simulink model "satellite_ADCS_detumbling_simulation_reaction_wheels"  (R2022b)
settings: Solver=FixedStepAuto  StartTime=t0  StopTime=T_o  FixedStep=0.1  RelTol=1e-9  AbsTol=1e-9
values from neighbouring files (symbols this model uses):
  A0 = Af    [satellite_ADCS_LEOP_simulation.m]
  a0 = [adx0 ady0 adz0 ax0 ay0 az0]    [satellite_ADCS_LEOP_simulation.m]
  A_sb_1 = [999.999999992226e-003    3.46376307675883e-006   -1.88420189887425e-006 ... (first row only)    [satellite_ADCS_LEOP_simulation.m]
  A_sb_2 = [999.999999948501e-003   -10.1488410044293e-006   -22.0178875132149e-012 ... (first row only)    [satellite_ADCS_LEOP_simulation.m]
  A_sb_3 = [999.999999975613e-003   -46.6812699606578e-012    6.98384920637069e-006 ... (first row only)    [satellite_ADCS_LEOP_simulation.m]
  Ac = [0 (1-Ky)*n 0 -Ky*n^2 0 0 ... (first row only)    [satellite_ADCS_LEOP_simulation.m]
  alphaG_0 = pi/1.5    (= 2.09439510239)    [satellite_ADCS_LEOP_simulation.m]
  ARW = [0 0; 1 0; 0 1]    [satellite_ADCS_LEOP_simulation.m]
  Bc = [J^-1; zeros(3,3)]    [satellite_ADCS_LEOP_simulation.m]
  Cc = [0 0 0 1 0 0 ... (first row only)    [satellite_ADCS_LEOP_simulation.m]
  Dc = zeros(3,3)    [satellite_ADCS_LEOP_simulation.m]
  E = 1    [satellite_ADCS_LEOP_simulation.m]
  F = 1e-3    (= 0.001)    [satellite_ADCS_LEOP_simulation.m]
  FOV = deg2rad(21.7)    [satellite_ADCS_LEOP_simulation.m]
  g_nm = S_matrix.*g_coefficients    [satellite_ADCS_LEOP_simulation.m]
  h_nm = S_matrix.*h_coefficients    [satellite_ADCS_LEOP_simulation.m]
  Irw = 80e-6    (= 8e-05)    [satellite_ADCS_LEOP_simulation.m]
  J = diag([Ix,Iy,Iz])    [satellite_ADCS_LEOP_simulation.m]
  J2 = 1.082e-3    (= 0.001082)    [satellite_ADCS_LEOP_simulation.m]
  K = lqry(SC,Qc,Rc)    [satellite_ADCS_LEOP_simulation.m]
  K_matrix = zeros(5,6)    [satellite_ADCS_LEOP_simulation.m]
  kep = [a e i OM om thf]    [satellite_ADCS_LEOP_simulation.m]
  L = Lt'    [satellite_ADCS_LEOP_simulation.m]
  LL = 1e-5    (= 1e-05)    [satellite_ADCS_LEOP_simulation.m]
  m = [0.37 0.32 0.28]    [satellite_ADCS_LEOP_simulation.m]
  mu = astroConstants(13)    [satellite_ADCS_LEOP_simulation.m]
  n = sqrt(mu/(a^3))    [satellite_ADCS_LEOP_simulation.m]
  n_sun = 2*pi/T_y    (= 1.99238499086e-07)    [satellite_ADCS_LEOP_simulation.m]
  omega_e = 2*pi/T_e    (= 7.27220521664e-05)    [satellite_ADCS_LEOP_simulation.m]
  P00 = 1    [satellite_ADCS_LEOP_simulation.m]
  pARW = pinv(ARW)    [satellite_ADCS_LEOP_simulation.m]
  pRRW = pinv(RRW)    [satellite_ADCS_LEOP_simulation.m]
  RRW = [R(:,3) R(:,6)]    [satellite_ADCS_LEOP_simulation.m]
  rt = astroConstants(23)    [satellite_ADCS_LEOP_simulation.m]
  S = S'    [satellite_ADCS_LEOP_simulation.m]
  sensor_noise = deg2rad(50/3600)    [satellite_ADCS_LEOP_simulation.m]
  sensor_sample_time = 1    [satellite_ADCS_LEOP_simulation.m]
  t0 = tf    (= 3200)    [satellite_ADCS_LEOP_simulation.m]
  T_o = 2*pi/n    [satellite_ADCS_LEOP_simulation.m]
  Te = 0.03    [satellite_ADCS_LEOP_simulation.m]
  Tp = [999.999926226686e-003    355.891478141766e-006   -144.526391847740e-006 ... (first row only)    [satellite_ADCS_LEOP_simulation.m]
  UL = 1e-4    (= 0.0001)    [satellite_ADCS_LEOP_simulation.m]
  w0 = wf    [satellite_ADCS_LEOP_simulation.m]
libraries: matrix_library x9, vrlib x3, sharedutil x2, aerolibutil x2
(part 1 of 3)
settings Model: Creator=user  LastModifiedBy=mutti
settings SolverCC: ZeroCrossAlgorithm=Adaptive
settings DebuggingCC: IgnoredZcDiagnostic=none  UnconnectedInputMsg=warning  UnconnectedOutputMsg=warning  UnconnectedLineMsg=warning
settings ModelReferenceCC: EnableRefExpFcnMdlSchedulingChecks=on
settings RTWCC: DLArmComputeVersion=19.05

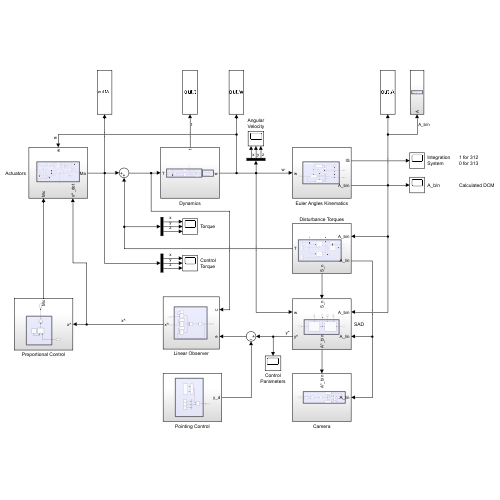
[thumbnail: Simulink's stored preview of the top-level diagram]
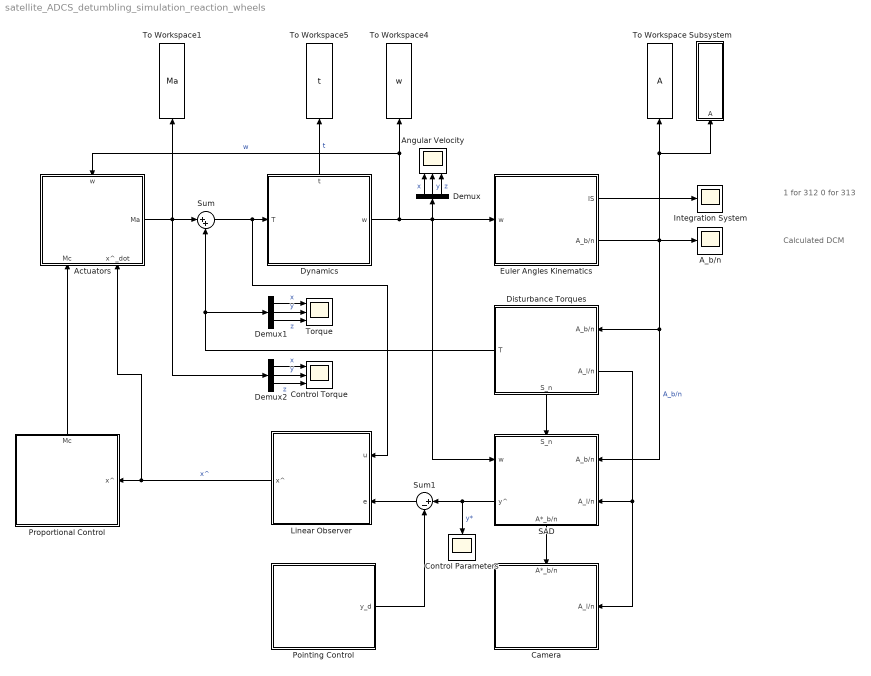
== system satellite_ADCS_detumbling_simulation_reaction_wheels ==
  note: Calculated DCM
  note: 1 for 312
      | 0 for 313
  A_b/n : Scope
  Actuators : Subsystem
      settings: PortSchema="{\"entries\":[{\"content\":{\"sides\":[{\"content\":{\"connectorIds\":[]},\"type\":\"ConnectorPlacement.EquallySpacedRectSide\",\"uuid\":\"a0a9569f-fefa-4f19-b459-3352d21c4e78\"},{\"content\":{\"connectorIds\":[\"Out1\"],\"side\":\"RIGHT\"},\"type\":\"ConnectorPlacement.EquallySpacedRectSide\",\"uuid\":\"2ed4db34-f6b5-4db4-9643-fbe8b2d4c52e\"},{\"content\":{\"connectorIds\":[\"In1\"],\"side\":\"TOP\"},\"type\":\"ConnectorPlacement.EquallySpacedRectSide\",\"uuid\":\"588bf8a5-5948-433a-b01f-23f1c7f2767b\"},{\"content\":{\"connectorIds\":[\"In2\",\"In3\"],\"side\":\"BOTTOM\"},\"type\":\"ConnectorPlacement.EquallySpacedRectSide\",\"uuid\":\"74bf1768-e871-4852-aab7-12511eae1523\"}]},\"type\":\"ConnectorPlacement.EquallySpacedConnector\",\"uuid\":\"47f49737-05d9-4a9e-a53b-421c1f23d8ed\"}],\"packageUris\":[\"http://schema.mathworks.com/mf0/Connector/R2020b\"],\"version\":\"1.0\"}"
  Angular Velocity : Scope  NumInputPorts=3
  Camera : Subsystem
      settings: PortSchema="{\"entries\":[{\"content\":{\"sides\":[{\"content\":{\"connectorIds\":[]},\"type\":\"ConnectorPlacement.EquallySpacedRectSide\",\"uuid\":\"e0342758-6e9b-40ff-85f6-f597544b67fd\"},{\"content\":{\"connectorIds\":[\"In2\"],\"side\":\"RIGHT\"},\"type\":\"ConnectorPlacement.EquallySpacedRectSide\",\"uuid\":\"f1e7fd7c-e0fe-4b5c-979b-e210999abd13\"},{\"content\":{\"connectorIds\":[\"In1\"],\"side\":\"TOP\"},\"type\":\"ConnectorPlacement.EquallySpacedRectSide\",\"uuid\":\"d086a2d5-2a33-45d1-927e-e3365679e422\"}]},\"type\":\"ConnectorPlacement.EquallySpacedConnector\",\"uuid\":\"0e539776-2a37-4829-8b62-d03ad8f161c7\"}],\"packageUris\":[\"http://schema.mathworks.com/mf0/Connector/R2020b\"],\"version\":\"1.0\"}"
  Control Parameters : Scope
  Control Torque : Scope  NumInputPorts=3
  Demux : Demux  Outputs=3
  Demux1 : Demux  Outputs=3
  Demux2 : Demux  Outputs=3
  Disturbance Torques : Subsystem
      settings: PortSchema="{\"entries\":[{\"content\":{\"sides\":[{\"content\":{\"connectorIds\":[\"In1\",\"Out3\"]},\"type\":\"ConnectorPlacement.EquallySpacedRectSide\",\"uuid\":\"d8dbad7b-a4da-4329-8f6c-994df882582d\"},{\"content\":{\"connectorIds\":[\"Out1\"],\"side\":\"RIGHT\"},\"type\":\"ConnectorPlacement.EquallySpacedRectSide\",\"uuid\":\"71b72684-f507-4d89-9cb7-6797f090e973\"},{\"content\":{\"connectorIds\":[],\"side\":\"TOP\"},\"type\":\"ConnectorPlacement.EquallySpacedRectSide\",\"uuid\":\"b8ec4cb7-c2c1-48ba-a366-4a3a04a391cc\"},{\"content\":{\"connectorIds\":[\"Out2\"],\"side\":\"BOTTOM\"},\"type\":\"ConnectorPlacement.EquallySpacedRectSide\",\"uuid\":\"004aaa39-3140-479a-bdad-82dbff681ba0\"}]},\"type\":\"ConnectorPlacement.EquallySpacedConnector\",\"uuid\":\"ddc3df03-ef2b-49f6-b8e4-ebb938f47d6c\"}],\"packageUris\":[\"http://schema.mathworks.com/mf0/Connector/R2020b\"],\"version\":\"1.0\"}"
  Dynamics : Subsystem
      settings: PortSchema="{\"entries\":[{\"content\":{\"sides\":[{\"content\":{\"connectorIds\":[\"In1\"]},\"type\":\"ConnectorPlacement.EquallySpacedRectSide\",\"uuid\":\"e7b72fe9-4828-4452-a73c-2aaa17307ac7\"},{\"content\":{\"connectorIds\":[\"Out1\"],\"side\":\"RIGHT\"},\"type\":\"ConnectorPlacement.EquallySpacedRectSide\",\"uuid\":\"e84d647a-1118-4c7e-bc5c-dae15a42ae60\"},{\"content\":{\"connectorIds\":[\"Out2\"],\"side\":\"TOP\"},\"type\":\"ConnectorPlacement.EquallySpacedRectSide\",\"uuid\":\"569f1d88-6323-45de-8d4a-941f3a02b2f9\"}]},\"type\":\"ConnectorPlacement.EquallySpacedConnector\",\"uuid\":\"aa1e349e-a763-481c-95bf-6bf3ac91b468\"}],\"packageUris\":[\"http://schema.mathworks.com/mf0/Connector/R2020b\"],\"version\":\"1.0\"}"
  Euler Angles Kinematics : Subsystem
  Integration System : Scope
  Linear Observer : Subsystem
  Pointing Control : Subsystem
  Proportional Control : Subsystem
      settings: PortSchema="{\"entries\":[{\"content\":{\"sides\":[{\"content\":{\"connectorIds\":[]},\"type\":\"ConnectorPlacement.EquallySpacedRectSide\",\"uuid\":\"b55cb1e2-f8e3-4e70-b41f-1afef80754b6\"},{\"content\":{\"connectorIds\":[\"In1\"],\"side\":\"RIGHT\"},\"type\":\"ConnectorPlacement.EquallySpacedRectSide\",\"uuid\":\"efac30e1-3844-4796-88a6-2f6a0b4b5a1e\"},{\"content\":{\"connectorIds\":[\"Out1\"],\"side\":\"TOP\"},\"type\":\"ConnectorPlacement.EquallySpacedRectSide\",\"uuid\":\"03ef4747-b6ea-4759-bd62-b95959aa7b4f\"}]},\"type\":\"ConnectorPlacement.EquallySpacedConnector\",\"uuid\":\"ca8bc0e9-cee1-4f1e-ac68-a532e2ed0ced\"}],\"packageUris\":[\"http://schema.mathworks.com/mf0/Connector/R2020b\"],\"version\":\"1.0\"}"
  SAD : Subsystem
      settings: PortSchema="{\"entries\":[{\"content\":{\"sides\":[{\"content\":{\"connectorIds\":[\"In1\",\"Out2\"]},\"type\":\"ConnectorPlacement.EquallySpacedRectSide\",\"uuid\":\"4f277e89-d200-473f-af52-c9445afe2970\"},{\"content\":{\"connectorIds\":[\"In3\",\"In4\"],\"side\":\"RIGHT\"},\"type\":\"ConnectorPlacement.EquallySpacedRectSide\",\"uuid\":\"94984762-2a8a-4315-bbca-0599c057d803\"},{\"content\":{\"connectorIds\":[\"In2\"],\"side\":\"TOP\"},\"type\":\"ConnectorPlacement.EquallySpacedRectSide\",\"uuid\":\"7e735617-ddb2-4178-9919-23d54f0f435d\"},{\"content\":{\"connectorIds\":[\"Out1\"],\"side\":\"BOTTOM\"},\"type\":\"ConnectorPlacement.EquallySpacedRectSide\",\"uuid\":\"8618ad89-dd0b-4af6-bdfc-ad96cd4377bc\"}]},\"type\":\"ConnectorPlacement.EquallySpacedConnector\",\"uuid\":\"e5f6a8ae-b3bf-403b-9441-c8c91592678e\"}],\"packageUris\":[\"http://schema.mathworks.com/mf0/Connector/R2020b\"],\"version\":\"1.0\"}"
  Subsystem : Subsystem
  Sum : Sum  Inputs=|++
  Sum1 : Sum  Inputs=|+-
  To Workspace : ToWorkspace  VariableName=A  SampleTime=-1
  To Workspace1 : ToWorkspace  VariableName=Ma  SampleTime=-1
  To Workspace4 : ToWorkspace  VariableName=w  SampleTime=-1
  To Workspace5 : ToWorkspace  VariableName=t  SampleTime=-1
  Torque : Scope  NumInputPorts=3
  wires:
  Dynamics/2(t) -> To Workspace5/1  "t"
  Dynamics/1(w) -> Demux/1, SAD/1(w), Euler Angles Kinematics/1(w), To Workspace4/1, Actuators/1(w)  "w"
  Euler Angles Kinematics/2(A_b/n) -> SAD/3(A_b/n), Disturbance Torques/1(A_b/n), A_b/n/1, Subsystem/1(A), To Workspace/1  "A_b/n"
  Demux/3 -> Angular Velocity/3  "z"
  Demux/2 -> Angular Velocity/2  "y"
  Demux/1 -> Angular Velocity/1  "x"
  Disturbance Torques/1(T) -> Sum/2, Demux1/1
  Demux1/1 -> Torque/1  "x"
  Demux1/3 -> Torque/3  "z"
  Demux1/2 -> Torque/2  "y"
  Euler Angles Kinematics/1(IS) -> Integration System/1
  Disturbance Torques/3(A_l/n) -> Camera/2(A_l/n), SAD/4(A_l/n)
  Sum/1 -> Linear Observer/1(u), Dynamics/1(T)
  SAD/2(y^) -> Sum1/1, Control Parameters/1  "y*"
  Disturbance Torques/2(S_n) -> SAD/2(S_n)
  Linear Observer/1(x^) -> Actuators/3(x^_dot), Proportional Control/1(x^)  "x^"
  Demux2/2 -> Control Torque/2  "y"
  Demux2/3 -> Control Torque/3  "z"
  Demux2/1 -> Control Torque/1  "x"
  Actuators/1(Ma) -> Demux2/1, Sum/1, To Workspace1/1
  SAD/1(A*_b/n) -> Camera/1(A*_b/n)
  Sum1/1 -> Linear Observer/2(e)
  Pointing Control/1(y_d) -> Sum1/2
  Proportional Control/1(Mc) -> Actuators/2(Mc)

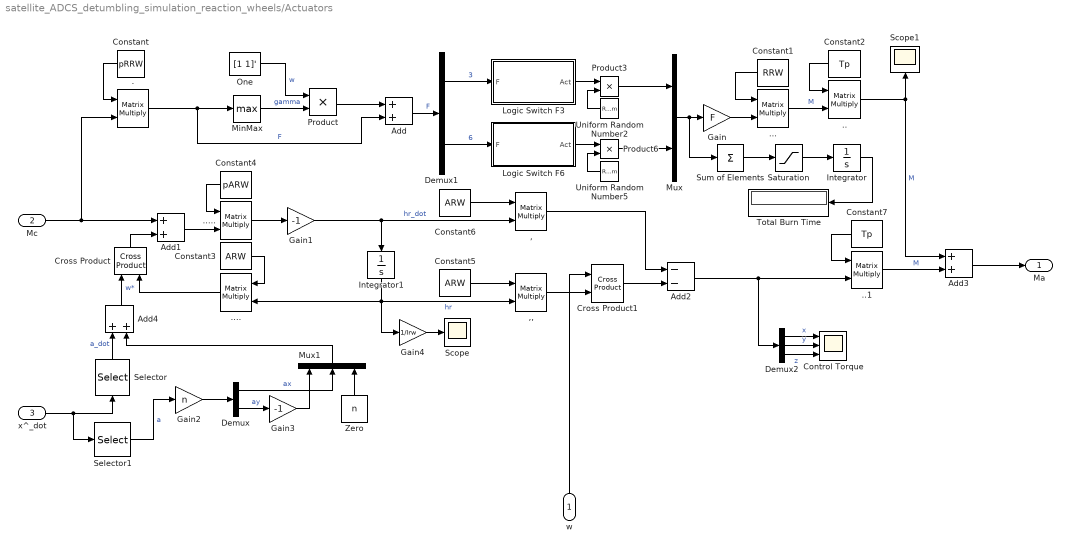
== system satellite_ADCS_detumbling_simulation_reaction_wheels/Actuators ==
  w : Inport
  Mc : Inport  Port=2
  x^_dot : Inport  Port=3
  , : Product  Multiplication=Matrix(*)
  ,, : Product  Multiplication=Matrix(*)
  . : Product  Multiplication=Matrix(*)
  .. : Product  Multiplication=Matrix(*)
  ... : Product  Multiplication=Matrix(*)
  .... : Product  Multiplication=Matrix(*)
  ..... : Product  Multiplication=Matrix(*)
  ..1 : Product  Multiplication=Matrix(*)
  Add{,1,3..4} (4 alike) : Sum
  Add2 : Sum  Inputs=--
  Constant : Constant  Value=pRRW
  Constant1 : Constant  Value=RRW
  Constant2 : Constant  Value=Tp
  Constant3 : Constant  Value=ARW
  Constant4 : Constant  Value=pARW
  Constant5 : Constant  Value=ARW
  Constant6 : Constant  Value=ARW
  Constant7 : Constant  Value=Tp
  Control Torque : Scope  NumInputPorts=3
  Cross Product : matrix_library/Cross Product
  Cross Product1 : matrix_library/Cross Product
  Demux : Demux  Outputs=2
  Demux1 : Demux  Outputs=2
  Demux2 : Demux  Outputs=3
  Gain : Gain  Gain=F
  Gain1 : Gain  Gain=-1
  Gain2 : Gain  Gain=n
  Gain3 : Gain  Gain=-1
  Gain4 : Gain  Gain=1/Irw
  Integrator : Integrator
  Integrator1 : Integrator  InitialCondition=[0 0]'
  Logic Switch F3 : Subsystem
  Logic Switch F6 : Subsystem
  MinMax : MinMax  Function=max
  Mux : Mux  Inputs=2
  Mux1 : Mux  Inputs=3
  One : Constant  Value=[1 1]'  OutDataTypeStr=Inherit: Inherit via back propagation
  Product : Product
  Product3 : Product
  Product6 : Product
  Saturation : Saturate  UpperLimit=1  LowerLimit=0
  Scope : Scope
  Scope1 : Scope
  Selector : Selector  InputPortWidth=6  IndexOptions=Index vector (dialog)  Indices=[1 2 3]  OutputSizes=1
  Selector1 : Selector  InputPortWidth=6  IndexOptions=Index vector (dialog)  Indices=[4 5]  OutputSizes=1
  Sum of Elements : Sum  Inputs=+
  Total Burn Time : Display
  Uniform Random Number2 : UniformRandomNumber  Minimum=1-Te  Maximum=1+Te  SampleTime=sensor_sample_time
  Uniform Random Number5 : UniformRandomNumber  Minimum=1-Te  Maximum=1+Te  SampleTime=sensor_sample_time
  Zero : Constant  Value=n  OutDataTypeStr=Inherit: Inherit via back propagation
  Ma : Outport
  wires:
  Gain4/1 -> Scope/1
  ..1/1 -> Add3/2  "M"
  Constant7/1 -> ..1/1
  Demux2/1 -> Control Torque/1  "x"
  Add2/1 -> ..1/2, Demux2/1
  Demux2/2 -> Control Torque/2  "y"
  Demux2/3 -> Control Torque/3  "z"
  Mux1/1 -> Add4/2
  Add4/1 -> Cross Product/1  "w*"
  Zero/1 -> Mux1/3
  Gain3/1 -> Mux1/1
  x^_dot/1 -> Selector1/1, Selector/1
  Gain2/1 -> Demux/1
  Demux/2 -> Gain3/1  "ay"
  Demux/1 -> Mux1/2  "ax"
  Selector1/1 -> Gain2/1  "a"
  Selector/1 -> Add4/1  "a_dot"
  Add3/1 -> Ma/1
  ,/1 -> Add2/1
  Cross Product1/1 -> Add2/2
  Constant6/1 -> ,/1
  ,,/1 -> Cross Product1/2
  Constant5/1 -> ,,/1
  w/1 -> Cross Product1/1
  Cross Product/1 -> Add1/2
  ..../1 -> Cross Product/2
  Gain1/1 -> ,/2, Integrator1/1  "hr_dot"
  ...../1 -> Gain1/1
  Constant4/1 -> ...../1
  Add1/1 -> ...../2
  Constant3/1 -> ..../1
  Integrator1/1 -> ..../2, ,,/2, Gain4/1  "hr"
  Constant2/1 -> ../1
  Constant1/1 -> .../1
  .../1 -> ../2  "M"
  Product3/1 -> Mux/1
  Product6/1 -> Mux/2
  Uniform Random Number5/1 -> Product6/2
  Uniform Random Number2/1 -> Product3/2
  Integrator/1 -> Total Burn Time/1
  Saturation/1 -> Integrator/1
  Sum of Elements/1 -> Saturation/1
  Gain/1 -> .../2
  Mux/1 -> Gain/1, Sum of Elements/1
  Logic Switch F3/1(Act) -> Product3/1
  Logic Switch F6/1(Act) -> Product6/1
  ../1 -> Scope1/1, Add3/1  "M"
  Demux1/1 -> Logic Switch F3/1(F)  "3"
  Demux1/2 -> Logic Switch F6/1(F)  "6"
  Add/1 -> Demux1/1  "F"
  Product/1 -> Add/1
  One/1 -> Product/1  "w"
  MinMax/1 -> Product/2  "gamma"
  ./1 -> Add/2, MinMax/1  "F"
  Mc/1 -> ./2, Add1/1
  Constant/1 -> ./1

== system satellite_ADCS_detumbling_simulation_reaction_wheels/Camera ==
  A*_b/n : Inport
  A_l/n : Inport  Port=2
  . : Product  Multiplication=Matrix(*)
  Asin : Trigonometry  Operator=asin
  Atan2 : Trigonometry  Operator=atan2
  Demux : Demux  Outputs=3
  Gain : Gain  Gain=-1
  Reshape : Reshape
  Reshape1 : Reshape
  Scope : Scope  NumInputPorts=2
  Selector : Selector  NumberOfDimensions=2  InputPortWidth=3  IndexOptions=Index vector (dialog),Index vector (dialog)  Indices=[1 2 3],1  OutputSizes=1,1
  To Workspace : ToWorkspace  VariableName=lat_lambda  SampleTime=-1
      settings: Save2DSignal=2-D array (concatenate along first dimension)
  To Workspace1 : ToWorkspace  VariableName=long_phi  SampleTime=-1
      settings: Save2DSignal=2-D array (concatenate along first dimension)
  Transpose : Math  Operator=transpose
  wires:
  A_l/n/1 -> Transpose/1
  A*_b/n/1 -> ./1
  ./1 -> Selector/1  "A_b/l"
  Selector/1 -> Demux/1  "x_b/l"
  Demux/3 -> Asin/1
  Asin/1 -> Scope/2, Reshape/1  "lat lambda"
  Demux/2 -> Atan2/1
  Demux/1 -> Atan2/2
  Atan2/1 -> Gain/1
  Transpose/1 -> ./2  "A_n/l"
  Gain/1 -> Scope/1, Reshape1/1  "long phi"
  Reshape/1 -> To Workspace/1
  Reshape1/1 -> To Workspace1/1

== system satellite_ADCS_detumbling_simulation_reaction_wheels/Disturbance Torques ==
  A_b/n : Inport
  Attitude Error : Subsystem
      settings: PortSchema="{\"entries\":[{\"content\":{\"sides\":[{\"content\":{\"connectorIds\":[\"In1\",\"Out1\"]},\"type\":\"ConnectorPlacement.EquallySpacedRectSide\",\"uuid\":\"42b76f21-72ca-4a81-86e8-c766a84eaf13\"},{\"content\":{\"connectorIds\":[],\"side\":\"RIGHT\"},\"type\":\"ConnectorPlacement.EquallySpacedRectSide\",\"uuid\":\"045cfb84-697d-470f-9812-3dd1de7d9dae\"},{\"content\":{\"connectorIds\":[],\"side\":\"TOP\"},\"type\":\"ConnectorPlacement.EquallySpacedRectSide\",\"uuid\":\"bb53017d-cb0a-420c-8e45-e706475f7b71\"},{\"content\":{\"connectorIds\":[\"In2\"],\"side\":\"BOTTOM\"},\"type\":\"ConnectorPlacement.EquallySpacedRectSide\",\"uuid\":\"54ff18d1-a59a-458c-93f1-94e0d804cb2b\"}]},\"type\":\"ConnectorPlacement.EquallySpacedConnector\",\"uuid\":\"29a17c75-6caa-44fa-8f21-b7e933b3095b\"}],\"packageUris\":[\"http://schema.mathworks.com/mf0/Connector/R2020b\"],\"version\":\"1.0\"}"
  GG Torque : Scope
  GGT : Subsystem
      settings: PortSchema="{\"entries\":[{\"content\":{\"sides\":[{\"content\":{\"connectorIds\":[]},\"type\":\"ConnectorPlacement.EquallySpacedRectSide\",\"uuid\":\"c87f4cc9-8c7a-4c3d-b61f-c042856a7ec9\"},{\"content\":{\"connectorIds\":[],\"side\":\"RIGHT\"},\"type\":\"ConnectorPlacement.EquallySpacedRectSide\",\"uuid\":\"826a080d-b2ad-4022-8511-2b74ea66cdbd\"},{\"content\":{\"connectorIds\":[\"Out1\",\"Out2\"],\"side\":\"TOP\"},\"type\":\"ConnectorPlacement.EquallySpacedRectSide\",\"uuid\":\"8ee238e0-7e27-4db5-8615-50d5a9b316be\"}]},\"type\":\"ConnectorPlacement.EquallySpacedConnector\",\"uuid\":\"2b8a1979-eb0c-41eb-af64-c98b651bcc5f\"}],\"packageUris\":[\"http://schema.mathworks.com/mf0/Connector/R2020b\"],\"version\":\"1.0\"}"
  Gravity Gradient Torque : Subsystem
  Local S/C Frame : Subsystem
      settings: PortSchema="{\"entries\":[{\"content\":{\"sides\":[{\"content\":{\"connectorIds\":[\"Out3\"]},\"type\":\"ConnectorPlacement.EquallySpacedRectSide\",\"uuid\":\"19c66f1b-1487-47a5-99ee-e01045e7a130\"},{\"content\":{\"connectorIds\":[\"Out1\"],\"side\":\"RIGHT\"},\"type\":\"ConnectorPlacement.EquallySpacedRectSide\",\"uuid\":\"23994730-2288-4426-9fea-174ee661e5cc\"},{\"content\":{\"connectorIds\":[\"Out2\"],\"side\":\"TOP\"},\"type\":\"ConnectorPlacement.EquallySpacedRectSide\",\"uuid\":\"3f4149a4-c086-47bf-a88a-6d224e7bd6a7\"}]},\"type\":\"ConnectorPlacement.EquallySpacedConnector\",\"uuid\":\"51dfc929-23d9-4c12-9475-93fee38e7017\"}],\"packageUris\":[\"http://schema.mathworks.com/mf0/Connector/R2020b\"],\"version\":\"1.0\"}"
  MD Torque : Scope
  MDT : Subsystem
      settings: PortSchema="{\"entries\":[{\"content\":{\"sides\":[{\"content\":{\"connectorIds\":[]},\"type\":\"ConnectorPlacement.EquallySpacedRectSide\",\"uuid\":\"c87f4cc9-8c7a-4c3d-b61f-c042856a7ec9\"},{\"content\":{\"connectorIds\":[],\"side\":\"RIGHT\"},\"type\":\"ConnectorPlacement.EquallySpacedRectSide\",\"uuid\":\"826a080d-b2ad-4022-8511-2b74ea66cdbd\"},{\"content\":{\"connectorIds\":[\"Out1\",\"Out2\"],\"side\":\"TOP\"},\"type\":\"ConnectorPlacement.EquallySpacedRectSide\",\"uuid\":\"8ee238e0-7e27-4db5-8615-50d5a9b316be\"}]},\"type\":\"ConnectorPlacement.EquallySpacedConnector\",\"uuid\":\"2b8a1979-eb0c-41eb-af64-c98b651bcc5f\"}],\"packageUris\":[\"http://schema.mathworks.com/mf0/Connector/R2020b\"],\"version\":\"1.0\"}"
  Magnetic Disturbance Torque n5 : Subsystem
  Manual Switch : ManualSwitch
  Manual Switch2 : ManualSwitch
  Sum : Sum  Inputs=|++
  Sun Position : Scope
  To Workspace2 : ToWorkspace  VariableName=R  SampleTime=-1
  Torque : Scope
  T : Outport
  S_n : Outport  Port=2
  A_l/n : Outport  Port=3
  wires:
  Gravity Gradient Torque/1(T) -> GG Torque/1, Sum/2  "T"
  A_b/n/1 -> Magnetic Disturbance Torque n5/1(A_b/n), Attitude Error/1(A_b/n)
  Manual Switch2/1 -> Magnetic Disturbance Torque n5/Enable
  GGT/1(On) -> Manual Switch/1
  MDT/2(Off) -> Manual Switch2/2
  Manual Switch/1 -> Gravity Gradient Torque/Enable
  Local S/C Frame/1(r_n) -> Gravity Gradient Torque/2(r_n), To Workspace2/1, Magnetic Disturbance Torque n5/2(r_n)
  GGT/2(Off) -> Manual Switch/2
  Local S/C Frame/3(S_n) -> S_n/1, Sun Position/1
  MDT/1(On) -> Manual Switch2/1
  Sum/1 -> Torque/1, T/1
  Magnetic Disturbance Torque n5/1(T) -> Sum/1, MD Torque/1
  Local S/C Frame/2(A_l/n) -> A_l/n/1, Attitude Error/2(A_l/n)
  Attitude Error/1(A_b/l) -> Gravity Gradient Torque/1(A_b/l)

== system satellite_ADCS_detumbling_simulation_reaction_wheels/Dynamics ==
  note: Time Track
  note: S/C Dynamics
  T : Inport
  Add : Sum
  Clock : Clock
  Constant5 : Constant  Value=J
  Cross Product : matrix_library/Cross Product
  Diagonal Matrix Inversion : Subsystem
  Integrator : Integrator  InitialCondition=w0  WrappedStateUpperValue=2*pi  WrappedStateLowerValue=0
  Matrix Multiply : Product  Multiplication=Matrix(*)
  Matrix Multiply1 : Product  Multiplication=Matrix(*)
  w : Outport
  t : Outport  Port=2
  wires:
  Integrator/1 -> Matrix Multiply/2, w/1, Cross Product/2  "w"
  Constant5/1 -> Diagonal Matrix Inversion/1(J), Matrix Multiply/1
  Matrix Multiply/1 -> Cross Product/1
  T/1 -> Add/1  "T"
  Cross Product/1 -> Add/2  "Jw x w"
  Add/1 -> Matrix Multiply1/2
  Matrix Multiply1/1 -> Integrator/1  "w_dot"
  Clock/1 -> t/1
  Diagonal Matrix Inversion/1(J') -> Matrix Multiply1/1

== system satellite_ADCS_detumbling_simulation_reaction_wheels/Euler Angles Kinematics ==
  note: Singularity Triggered Kinematics
  w : Inport
  312 kin : Subsystem  TreatAsAtomicUnit=on
  313 kin : Subsystem  TreatAsAtomicUnit=on
  Delay : Delay  DelayLength=1  InitialCondition=1
  Determinant of 3x3 Matrix : sharedutil/Determinant of 3x3 Matrix  aMode=aMode
  Flip Check : Scope
  Initial Conditions : Subsystem
  Merge : Merge
  Merge1 : Merge
  NOT : Logic  Operator=NOT  AllPortsSameDT=off  OutDataTypeStr=boolean
  Orthogonality Check : Scope
  IS : Outport
  A_b/n : Outport  Port=2
  wires:
  Initial Conditions/1(E) -> 312 kin/Enable, NOT/1
  w/1 -> 313 kin/1(Input), 312 kin/1(w)
  Merge1/1 -> Determinant of 3x3 Matrix/1, A_b/n/1
  313 kin/2(E) -> Merge/2
  Merge/1 -> IS/1, Delay/1
  NOT/1 -> 313 kin/Enable
  Delay/1 -> Flip Check/1, Initial Conditions/1(S)
  312 kin/1(E) -> Merge/1
  312 kin/2(A) -> Merge1/1
  313 kin/1(A) -> Merge1/2
  Determinant of 3x3 Matrix/1 -> Orthogonality Check/1

== system satellite_ADCS_detumbling_simulation_reaction_wheels/Linear Observer ==
  u : Inport
  e : Inport  Port=2
  . : Product  Multiplication=Matrix(*)
  .. : Product  Multiplication=Matrix(*)
  ... : Product  Multiplication=Matrix(*)
  Add : Sum  Inputs=+++
  Constant : Constant  Value=L
  Constant1 : Constant  Value=Bc-L*Dc
  Constant2 : Constant  Value=Ac-L*Cc
  Integrator : Integrator  InitialCondition=a0
  x^ : Outport
  wires:
  e/1 -> ./2
  Constant/1 -> ./1
  u/1 -> ../2
  Constant1/1 -> ../1
  Constant2/1 -> .../1
  ./1 -> Add/1
  ../1 -> Add/2
  .../1 -> Add/3
  Add/1 -> Integrator/1  "x^_dot"
  Integrator/1 -> x^/1, .../2

== system satellite_ADCS_detumbling_simulation_reaction_wheels/Pointing Control ==
  Manual Control : Subsystem
      settings: PortSchema="{\"entries\":[{\"content\":{\"sides\":[{\"content\":{\"connectorIds\":[]},\"type\":\"ConnectorPlacement.EquallySpacedRectSide\",\"uuid\":\"c87f4cc9-8c7a-4c3d-b61f-c042856a7ec9\"},{\"content\":{\"connectorIds\":[],\"side\":\"RIGHT\"},\"type\":\"ConnectorPlacement.EquallySpacedRectSide\",\"uuid\":\"826a080d-b2ad-4022-8511-2b74ea66cdbd\"},{\"content\":{\"connectorIds\":[\"Out1\",\"Out2\"],\"side\":\"TOP\"},\"type\":\"ConnectorPlacement.EquallySpacedRectSide\",\"uuid\":\"8ee238e0-7e27-4db5-8615-50d5a9b316be\"}]},\"type\":\"ConnectorPlacement.EquallySpacedConnector\",\"uuid\":\"2b8a1979-eb0c-41eb-af64-c98b651bcc5f\"}],\"packageUris\":[\"http://schema.mathworks.com/mf0/Connector/R2020b\"],\"version\":\"1.0\"}"
  Manual Switch2 : ManualSwitch  CurrentSetting=0
  Mux : Mux  Inputs=3
  Product : Product
  Sine Wave : Sin  Amplitude=deg2rad(5)  Frequency=2*pi/T_o*8  SampleTime=0
  Sine Wave1 : Sin  Amplitude=deg2rad(12)  Frequency=2*pi/T_o*4  SampleTime=0
  Zero : Constant  Value=0  OutDataTypeStr=Inherit: Inherit via back propagation
  y_d : Outport
  wires:
  Mux/1 -> Product/2
  Zero/1 -> Mux/1
  Sine Wave/1 -> Mux/2
  Sine Wave1/1 -> Mux/3
  Manual Switch2/1 -> Product/1
  Manual Control/1(On) -> Manual Switch2/1
  Manual Control/2(Off) -> Manual Switch2/2
  Product/1 -> y_d/1

== system satellite_ADCS_detumbling_simulation_reaction_wheels/Proportional Control ==
  x^ : Inport
  . : Product  Multiplication=Matrix(*)
  Constant1 : Constant  Value=K
  Gain1 : Gain  Gain=-1
  Mc : Outport
  wires:
  Constant1/1 -> ./1
  x^/1 -> ./2
  ./1 -> Gain1/1  "u"
  Gain1/1 -> Mc/1

== system satellite_ADCS_detumbling_simulation_reaction_wheels/SAD ==
  w : Inport
  S_n : Inport  Port=2
  A_b/n : Inport  Port=3
  A_l/n : Inport  Port=4
  Attitude Determination : Subsystem
      settings: PortSchema="{\"entries\":[{\"content\":{\"sides\":[{\"content\":{\"connectorIds\":[\"Out1\"]},\"type\":\"ConnectorPlacement.EquallySpacedRectSide\",\"uuid\":\"0507266e-0c75-4cb2-99bc-34ebc9d3cde1\"},{\"content\":{\"connectorIds\":[\"In3\"],\"side\":\"RIGHT\"},\"type\":\"ConnectorPlacement.EquallySpacedRectSide\",\"uuid\":\"5a03a495-b095-40bf-8b9c-d2e1dd273ea9\"},{\"content\":{\"connectorIds\":[\"In1\",\"In2\"],\"side\":\"TOP\"},\"type\":\"ConnectorPlacement.EquallySpacedRectSide\",\"uuid\":\"ba817cf4-306f-4005-a0c6-f74e330936f6\"}]},\"type\":\"ConnectorPlacement.EquallySpacedConnector\",\"uuid\":\"5c804e99-5e54-4c88-bfff-7855a4e43f31\"}],\"packageUris\":[\"http://schema.mathworks.com/mf0/Connector/R2020b\"],\"version\":\"1.0\"}"
  Control Parameters : Subsystem
      settings: PortSchema="{\"entries\":[{\"content\":{\"sides\":[{\"content\":{\"connectorIds\":[\"Out1\"]},\"type\":\"ConnectorPlacement.EquallySpacedRectSide\",\"uuid\":\"4f277e89-d200-473f-af52-c9445afe2970\"},{\"content\":{\"connectorIds\":[\"In2\"],\"side\":\"RIGHT\"},\"type\":\"ConnectorPlacement.EquallySpacedRectSide\",\"uuid\":\"94984762-2a8a-4315-bbca-0599c057d803\"},{\"content\":{\"connectorIds\":[\"In1\"],\"side\":\"TOP\"},\"type\":\"ConnectorPlacement.EquallySpacedRectSide\",\"uuid\":\"7e735617-ddb2-4178-9919-23d54f0f435d\"}]},\"type\":\"ConnectorPlacement.EquallySpacedConnector\",\"uuid\":\"e5f6a8ae-b3bf-403b-9441-c8c91592678e\"}],\"packageUris\":[\"http://schema.mathworks.com/mf0/Connector/R2020b\"],\"version\":\"1.0\"}"
  A*_b/n : Outport
  y^ : Outport  Port=2
  wires:
  A_l/n/1 -> Control Parameters/1(A_l/n)
  A_b/n/1 -> Attitude Determination/3(A_b/n)
  S_n/1 -> Attitude Determination/1(S_n)
  Control Parameters/1(y^) -> y^/1
  Attitude Determination/1(A*_b/n) -> A*_b/n/1, Control Parameters/2(A*_b/n)
  w/1 -> Attitude Determination/2(w)

== system satellite_ADCS_detumbling_simulation_reaction_wheels/Subsystem ==
  note: b1 vector component of A
  note: b2 vector component of A
  note: b3 vector component of A
  A : Inport
  Selector : Selector  NumberOfDimensions=2  InputPortWidth=3  IndexOptions=Index vector (dialog),Index vector (dialog)  Indices=1,[1 2 3]  OutputSizes=1,1
  Selector1 : Selector  NumberOfDimensions=2  InputPortWidth=3  IndexOptions=Index vector (dialog),Index vector (dialog)  Indices=2,[1 2 3]  OutputSizes=1,1
  Selector2 : Selector  NumberOfDimensions=2  InputPortWidth=3  IndexOptions=Index vector (dialog),Index vector (dialog)  Indices=3,[1 2 3]  OutputSizes=1,1
  To Workspace : ToWorkspace  VariableName=bu  SampleTime=-1
  To Workspace1 : ToWorkspace  VariableName=bv  SampleTime=-1
  To Workspace2 : ToWorkspace  VariableName=bw  SampleTime=-1
  wires:
  A/1 -> Selector2/1, Selector/1, Selector1/1
  Selector/1 -> To Workspace/1
  Selector1/1 -> To Workspace1/1
  Selector2/1 -> To Workspace2/1

== system satellite_ADCS_detumbling_simulation_reaction_wheels/Actuators/Logic Switch F3 ==
  F : Inport
  Clock : Clock
  Delay : Delay  DelayLength=1
  Enabled Subsystem : Subsystem  TreatAsAtomicUnit=on
  Enabled Subsystem1 : Subsystem  TreatAsAtomicUnit=on
  GreaterThan : RelationalOperator  OutDataTypeStr=boolean  RndMeth=Simplest  InputSameDT=off
  Merge : Merge
  Merge1 : Merge
  NOT : Logic  Operator=NOT  AllPortsSameDT=off  OutDataTypeStr=boolean
  Scope1 : Scope
  Switch : Switch  Criteria=u2 > Threshold  SaturateOnIntegerOverflow=off  InputSameDT=off
  UL : Constant  Value=UL  OutDataTypeStr=Inherit: Inherit via back propagation
  Act : Outport
  wires:
  Merge/1 -> Delay/1
  GreaterThan/1 -> Switch/3
  UL/1 -> GreaterThan/2
  Merge1/1 -> Act/1
  Enabled Subsystem1/2(y) -> Merge1/2
  Switch/1 -> NOT/1, Enabled Subsystem/Enable
  Delay/1 -> Scope1/1, Switch/1
  Clock/1 -> Switch/2
  NOT/1 -> Enabled Subsystem1/Enable
  F/1 -> Enabled Subsystem/1(In1), Enabled Subsystem1/1(In1), GreaterThan/1
  Enabled Subsystem/2(y) -> Merge1/1
  Enabled Subsystem1/1(e) -> Merge/2
  Enabled Subsystem/1(e) -> Merge/1

== system satellite_ADCS_detumbling_simulation_reaction_wheels/Actuators/Logic Switch F6 ==
  F : Inport
  Clock : Clock
  Delay : Delay  DelayLength=1
  Enabled Subsystem : Subsystem  TreatAsAtomicUnit=on
  Enabled Subsystem1 : Subsystem  TreatAsAtomicUnit=on
  GreaterThan : RelationalOperator  OutDataTypeStr=boolean  RndMeth=Simplest  InputSameDT=off
  Merge : Merge
  Merge1 : Merge
  NOT : Logic  Operator=NOT  AllPortsSameDT=off  OutDataTypeStr=boolean
  Scope1 : Scope
  Switch : Switch  Criteria=u2 > Threshold  SaturateOnIntegerOverflow=off  InputSameDT=off
  UL : Constant  Value=UL  OutDataTypeStr=Inherit: Inherit via back propagation
  Act : Outport
  wires:
  Enabled Subsystem/1(e) -> Merge/1
  Enabled Subsystem1/1(e) -> Merge/2
  Enabled Subsystem/2(y) -> Merge1/1
  F/1 -> GreaterThan/1, Enabled Subsystem1/1(In1), Enabled Subsystem/1(In1)
  NOT/1 -> Enabled Subsystem1/Enable
  Clock/1 -> Switch/2
  Delay/1 -> Switch/1, Scope1/1
  Switch/1 -> Enabled Subsystem/Enable, NOT/1
  Enabled Subsystem1/2(y) -> Merge1/2
  Merge1/1 -> Act/1
  UL/1 -> GreaterThan/2
  GreaterThan/1 -> Switch/3
  Merge/1 -> Delay/1

== system satellite_ADCS_detumbling_simulation_reaction_wheels/Disturbance Torques/Attitude Error ==
  A_b/n : Inport
  A_l/n : Inport  Port=2
  Matrix Multiply1 : Product  Multiplication=Matrix(*)
  Transpose : Math  Operator=transpose
  A_b/l : Outport
  wires:
  Transpose/1 -> Matrix Multiply1/2  "A_n/l"
  A_l/n/1 -> Transpose/1
  A_b/n/1 -> Matrix Multiply1/1
  Matrix Multiply1/1 -> A_b/l/1

== system satellite_ADCS_detumbling_simulation_reaction_wheels/Disturbance Torques/GGT ==
  Constant : Constant
  Constant1 : Constant  Value=0
  On : Outport
  Off : Outport  Port=2
  wires:
  Constant/1 -> On/1
  Constant1/1 -> Off/1

== system satellite_ADCS_detumbling_simulation_reaction_wheels/Disturbance Torques/Gravity Gradient Torque ==
  note: this builds up error
  note: Gravity Gradient Perturbation Torque
  A_b/l : Inport
  r_n : Inport  Port=2
  Enable : EnablePort
  Attitude Error Matrix : Scope
  Constant : Constant  Value=mu
  Constant1 : Constant  Value=-3
  Constant5 : Constant  Value=J
  Cross Product1 : matrix_library/Cross Product
  Dot Product5 : DotProduct  OutDataTypeStr=Inherit: Inherit via internal rule
  Gain : Gain  Gain=3
  Gravitational Torque Check : Scope
  Matrix Multiply2 : Product  Multiplication=Matrix(*)
  Power : Math  Operator=pow
  Product : Product
  Product1 : Product
  Reshape : Reshape
  Selector : Selector  NumberOfDimensions=2  InputPortWidth=3  IndexOptions=Index vector (dialog),Index vector (dialog)  Indices=[1 2 3],1  OutputSizes=1,1
  Sqrt3 : Sqrt
  T : Outport
  wires:
  A_b/l/1 -> Selector/1, Attitude Error Matrix/1  "A_b/l"
  Selector/1 -> Cross Product1/1, Matrix Multiply2/2  "c"
  Matrix Multiply2/1 -> Cross Product1/2  "Jc"
  Cross Product1/1 -> Product1/1
  Constant5/1 -> Matrix Multiply2/1
  Product1/1 -> Gravitational Torque Check/1, Reshape/1
  Reshape/1 -> T/1
  Constant1/1 -> Power/2
  Power/1 -> Product/1
  Constant/1 -> Product/2
  Product/1 -> Gain/1
  Gain/1 -> Product1/2
  r_n/1 -> Dot Product5/1, Dot Product5/2  "r_n"
  Sqrt3/1 -> Power/1  "r"
  Dot Product5/1 -> Sqrt3/1

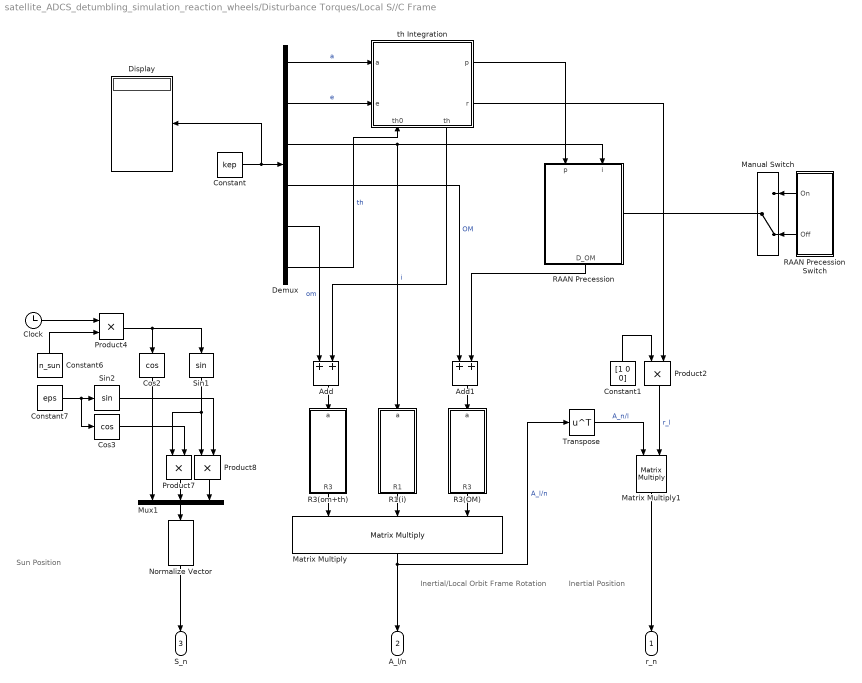
== system satellite_ADCS_detumbling_simulation_reaction_wheels/Disturbance Torques/Local S//C Frame ==
  note: Sun Position
  note: Inertial Position
  note: Inertial/Local Orbit Frame Rotation
  Add : Sum
  Add1 : Sum
  Clock : Clock
  Constant : Constant  Value=kep
  Constant1 : Constant  Value=[1 0 0]
  Constant6 : Constant  Value=n_sun
  Constant7 : Constant  Value=eps
  Cos2 : Trigonometry  Operator=cos
  Cos3 : Trigonometry  Operator=cos
  Demux : Demux  Outputs=6
  Display : Display
  Manual Switch : ManualSwitch  CurrentSetting=0
  Matrix Multiply : Product  Inputs=3  Multiplication=Matrix(*)
  Matrix Multiply1 : Product  Multiplication=Matrix(*)
  Mux1 : Mux  Inputs=3
  Normalize Vector : vrlib/Utilities/Normalize Vector  maxzero=0
  Product{2,4,7..8} (4 alike) : Product
  R1(i) : Subsystem
  R3(OM) : Subsystem
  R3(om+th) : Subsystem
  RAAN Precession : Subsystem
  RAAN Precession Switch : Subsystem
      settings: PortSchema="{\"entries\":[{\"content\":{\"sides\":[{\"content\":{\"connectorIds\":[]},\"type\":\"ConnectorPlacement.EquallySpacedRectSide\",\"uuid\":\"c87f4cc9-8c7a-4c3d-b61f-c042856a7ec9\"},{\"content\":{\"connectorIds\":[],\"side\":\"RIGHT\"},\"type\":\"ConnectorPlacement.EquallySpacedRectSide\",\"uuid\":\"826a080d-b2ad-4022-8511-2b74ea66cdbd\"},{\"content\":{\"connectorIds\":[\"Out1\",\"Out2\"],\"side\":\"TOP\"},\"type\":\"ConnectorPlacement.EquallySpacedRectSide\",\"uuid\":\"8ee238e0-7e27-4db5-8615-50d5a9b316be\"}]},\"type\":\"ConnectorPlacement.EquallySpacedConnector\",\"uuid\":\"2b8a1979-eb0c-41eb-af64-c98b651bcc5f\"}],\"packageUris\":[\"http://schema.mathworks.com/mf0/Connector/R2020b\"],\"version\":\"1.0\"}"
  Sin1 : Trigonometry
  Sin2 : Trigonometry
  Transpose : Math  Operator=transpose
  th Integration : Subsystem
      settings: PortSchema="{\"entries\":[{\"content\":{\"sides\":[{\"content\":{\"connectorIds\":[\"In1\",\"In2\"]},\"type\":\"ConnectorPlacement.EquallySpacedRectSide\",\"uuid\":\"334afb3e-b800-40ec-9197-fa5f68d698bb\"},{\"content\":{\"connectorIds\":[\"Out1\",\"Out2\"],\"side\":\"RIGHT\"},\"type\":\"ConnectorPlacement.EquallySpacedRectSide\",\"uuid\":\"abbffafe-b146-47e8-9f47-ef68c6093964\"},{\"content\":{\"connectorIds\":[],\"side\":\"TOP\"},\"type\":\"ConnectorPlacement.EquallySpacedRectSide\",\"uuid\":\"572a075b-4779-4b9c-a1c3-66ef8ad6430c\"},{\"content\":{\"connectorIds\":[\"In3\",\"Out3\"],\"side\":\"BOTTOM\"},\"type\":\"ConnectorPlacement.EquallySpacedRectSide\",\"uuid\":\"22d8f220-9523-4104-bc3a-d052975615ec\"}]},\"type\":\"ConnectorPlacement.EquallySpacedConnector\",\"uuid\":\"7f3f56c6-e778-456f-ad48-e4d4eca130ec\"}],\"packageUris\":[\"http://schema.mathworks.com/mf0/Connector/R2020b\"],\"version\":\"1.0\"}"
  r_n : Outport
  A_l/n : Outport  Port=2
  S_n : Outport  Port=3
  wires:
  Constant/1 -> Display/1, Demux/1
  Demux/3 -> RAAN Precession/2(i), R1(i)/1(a)  "i"
  Demux/4 -> Add1/1  "OM"
  Demux/5 -> Add/1  "om"
  Demux/1 -> th Integration/1(a)  "a"
  Demux/2 -> th Integration/2(e)  "e"
  Add/1 -> R3(om+th)/1(a)
  R3(om+th)/1(R3) -> Matrix Multiply/1
  R1(i)/1(R1) -> Matrix Multiply/2
  R3(OM)/1(R3) -> Matrix Multiply/3
  Transpose/1 -> Matrix Multiply1/1  "A_n/l"
  Matrix Multiply/1 -> Transpose/1, A_l/n/1  "A_l/n"
  Constant1/1 -> Product2/1
  Matrix Multiply1/1 -> r_n/1
  Product2/1 -> Matrix Multiply1/2  "r_l"
  Clock/1 -> Product4/1
  Constant6/1 -> Product4/2
  Product4/1 -> Sin1/1, Cos2/1
  Constant7/1 -> Cos3/1, Sin2/1
  Product8/1 -> Mux1/3
  Cos2/1 -> Mux1/1
  Product7/1 -> Mux1/2
  Sin1/1 -> Product8/1, Product7/1
  Cos3/1 -> Product7/2
  Sin2/1 -> Product8/2
  Mux1/1 -> Normalize Vector/1
  Normalize Vector/1 -> S_n/1
  Demux/6 -> th Integration/3(th0)  "th"
  Add1/1 -> R3(OM)/1(a)
  th Integration/2(r) -> Product2/2
  th Integration/3(th) -> Add/2
  th Integration/1(p) -> RAAN Precession/1(p)
  RAAN Precession/1(D_OM) -> Add1/2
  Manual Switch/1 -> RAAN Precession/Enable
  RAAN Precession Switch/1(Off) -> Manual Switch/2
  RAAN Precession Switch/2(On) -> Manual Switch/1

== system satellite_ADCS_detumbling_simulation_reaction_wheels/Disturbance Torques/MDT ==
  Constant : Constant
  Constant1 : Constant  Value=0
  On : Outport
  Off : Outport  Port=2
  wires:
  Constant/1 -> On/1
  Constant1/1 -> Off/1

== system satellite_ADCS_detumbling_simulation_reaction_wheels/Disturbance Torques/Magnetic Disturbance Torque n5 ==
  A_b/n : Inport
  r_n : Inport  Port=2
  Enable : EnablePort
  Constant3 : Constant  Value=m
  Cross Product : matrix_library/Cross Product
  Matrix Multiply : Product  Multiplication=Matrix(*)
  P and dP matrices : Subsystem
      settings: PortSchema="{\"entries\":[{\"content\":{\"sides\":[{\"content\":{\"connectorIds\":[]},\"type\":\"ConnectorPlacement.EquallySpacedRectSide\",\"uuid\":\"dab89660-b1ab-40c8-8b5f-10cb6b820ab4\"},{\"content\":{\"connectorIds\":[\"Out1\",\"Out2\"],\"side\":\"RIGHT\"},\"type\":\"ConnectorPlacement.EquallySpacedRectSide\",\"uuid\":\"7221400e-397e-409c-989a-99e2208831b4\"},{\"content\":{\"connectorIds\":[],\"side\":\"TOP\"},\"type\":\"ConnectorPlacement.EquallySpacedRectSide\",\"uuid\":\"eb5148c0-c1a9-4373-ad53-1b0d9d21f5e7\"},{\"content\":{\"connectorIds\":[\"In1\"],\"side\":\"BOTTOM\"},\"type\":\"ConnectorPlacement.EquallySpacedRectSide\",\"uuid\":\"c3f7c62b-4c65-42d2-a346-91e5251d2beb\"}]},\"type\":\"ConnectorPlacement.EquallySpacedConnector\",\"uuid\":\"22134191-a178-4a2a-a656-d39bf24db322\"}],\"packageUris\":[\"http://schema.mathworks.com/mf0/Connector/R2020b\"],\"version\":\"1.0\"}"
  Subsystem : Subsystem
      settings: PortSchema="{\"entries\":[{\"content\":{\"sides\":[{\"content\":{\"connectorIds\":[\"In1\"]},\"type\":\"ConnectorPlacement.EquallySpacedRectSide\",\"uuid\":\"b7806037-f1a8-4646-8130-063c6bc284ea\"},{\"content\":{\"connectorIds\":[\"Out1\",\"Out2\",\"Out3\",\"Out4\"],\"side\":\"RIGHT\"},\"type\":\"ConnectorPlacement.EquallySpacedRectSide\",\"uuid\":\"9dbabc58-60b6-45ae-a05b-7a245ad73091\"},{\"content\":{\"connectorIds\":[\"Out5\"],\"side\":\"TOP\"},\"type\":\"ConnectorPlacement.EquallySpacedRectSide\",\"uuid\":\"cacfcb4a-4f84-47f1-8789-145c966f7e80\"}]},\"type\":\"ConnectorPlacement.EquallySpacedConnector\",\"uuid\":\"a6632146-8bc8-4e1c-852e-afec4cb27c4d\"}],\"packageUris\":[\"http://schema.mathworks.com/mf0/Connector/R2020b\"],\"version\":\"1.0\"}"
  Subsystem1 : Subsystem
      settings: PortSchema="{\"entries\":[{\"content\":{\"sides\":[{\"content\":{\"connectorIds\":[\"In1\",\"In2\"]},\"type\":\"ConnectorPlacement.EquallySpacedRectSide\",\"uuid\":\"50e3ace2-2623-4246-9eef-f31fa2dd1d8a\"},{\"content\":{\"connectorIds\":[\"Out1\",\"Out2\",\"Out3\"],\"side\":\"RIGHT\"},\"type\":\"ConnectorPlacement.EquallySpacedRectSide\",\"uuid\":\"83d07770-a8f2-4dad-b423-cdd1e97b7dcd\"},{\"content\":{\"connectorIds\":[],\"side\":\"TOP\"},\"type\":\"ConnectorPlacement.EquallySpacedRectSide\",\"uuid\":\"df8fe2ed-c08c-48c6-abc8-f5a1f990ad2b\"},{\"content\":{\"connectorIds\":[\"In3\",\"In4\",\"In5\"],\"side\":\"BOTTOM\"},\"type\":\"ConnectorPlacement.EquallySpacedRectSide\",\"uuid\":\"71da06e9-1829-467d-8fff-f8f8dfe54512\"}]},\"type\":\"ConnectorPlacement.EquallySpacedConnector\",\"uuid\":\"d997f2a9-2378-49d1-921f-4989413f3125\"}],\"packageUris\":[\"http://schema.mathworks.com/mf0/Connector/R2020b\"],\"version\":\"1.0\"}"
  Subsystem5 : Subsystem
      settings: PortSchema="{\"entries\":[{\"content\":{\"sides\":[{\"content\":{\"connectorIds\":[\"In1\",\"In2\",\"In3\"]},\"type\":\"ConnectorPlacement.EquallySpacedRectSide\",\"uuid\":\"e24a2db4-8487-4955-87bf-3e800520ea69\"},{\"content\":{\"connectorIds\":[\"Out1\"],\"side\":\"RIGHT\"},\"type\":\"ConnectorPlacement.EquallySpacedRectSide\",\"uuid\":\"3755e0df-10e6-4862-a69b-331f0c086a8c\"},{\"content\":{\"connectorIds\":[],\"side\":\"TOP\"},\"type\":\"ConnectorPlacement.EquallySpacedRectSide\",\"uuid\":\"930661f6-ad92-4da4-b7ae-9811d8d77206\"},{\"content\":{\"connectorIds\":[\"In4\",\"In5\"],\"side\":\"BOTTOM\"},\"type\":\"ConnectorPlacement.EquallySpacedRectSide\",\"uuid\":\"f043b77a-ea9f-4eac-b602-153051b4efda\"}]},\"type\":\"ConnectorPlacement.EquallySpacedConnector\",\"uuid\":\"dd6959d8-c10a-4ac2-8395-1f077e6521ea\"}],\"packageUris\":[\"http://schema.mathworks.com/mf0/Connector/R2020b\"],\"version\":\"1.0\"}"
  Transpose1 : Math  Operator=transpose
  Transpose2 : Math  Operator=transpose
  T : Outport
  wires:
  Subsystem1/1(B_r) -> Subsystem5/1(Br)  "Br"
  Transpose2/1 -> Subsystem1/2(dP_matrix)  "dP_matrix"
  P and dP matrices/2(dP) -> Transpose2/1
  P and dP matrices/1(P) -> Transpose1/1
  Matrix Multiply/1 -> Cross Product/2  "b_b"
  Subsystem/1(r) -> Subsystem1/4(r)
  Subsystem1/3(B_phi) -> Subsystem5/3(Bphi)  "Bphi"
  Subsystem/3(RA) -> Subsystem5/4(RA)
  Transpose1/1 -> Subsystem1/1(P_matrix)  "P_matrix"
  Subsystem/4(DELTA) -> Subsystem5/5(DELTA)
  r_n/1 -> Subsystem/1(r_n)
  Constant3/1 -> Cross Product/1
  Subsystem1/2(B_theta) -> Subsystem5/2(Bth)  "Bth"
  Subsystem5/1(B_N) -> Matrix Multiply/2  "b_n"
  Subsystem/2(Longitude) -> Subsystem1/5(Longitude)
  Subsystem/5(Colatitude) -> Subsystem1/3(colatitude), P and dP matrices/1(colatitude)
  Cross Product/1 -> T/1
  A_b/n/1 -> Matrix Multiply/1

== system satellite_ADCS_detumbling_simulation_reaction_wheels/Dynamics/Diagonal Matrix Inversion ==
  note: Diagonal J Inversion
  J : Inport
  Constant : Constant  Value=-1
  Constant1 : Constant  Value=0
  Create 3x3 Matrix : sharedutil/Create 3x3 Matrix  aMode=aMode
  Power : Math  Operator=pow
  Power1 : Math  Operator=pow
  Power2 : Math  Operator=pow
  Selector : Selector  NumberOfDimensions=2  InputPortWidth=3  IndexOptions=Index vector (dialog),Index vector (dialog)  Indices=1,1  OutputSizes=1,1
  Selector1 : Selector  NumberOfDimensions=2  InputPortWidth=3  IndexOptions=Index vector (dialog),Index vector (dialog)  Indices=2,2  OutputSizes=1,1
  Selector2 : Selector  NumberOfDimensions=2  InputPortWidth=3  IndexOptions=Index vector (dialog),Index vector (dialog)  Indices=3,3  OutputSizes=1,1
  J' : Outport
  wires:
  J/1 -> Selector/1, Selector2/1, Selector1/1
  Create 3x3 Matrix/1 -> J'/1
  Selector/1 -> Power/1
  Selector1/1 -> Power1/1
  Selector2/1 -> Power2/1
  Constant/1 -> Power/2, Power1/2, Power2/2
  Power/1 -> Create 3x3 Matrix/1
  Power1/1 -> Create 3x3 Matrix/5
  Power2/1 -> Create 3x3 Matrix/9
  Constant1/1 -> Create 3x3 Matrix/8, Create 3x3 Matrix/2, Create 3x3 Matrix/3, Create 3x3 Matrix/4, Create 3x3 Matrix/6, Create 3x3 Matrix/7

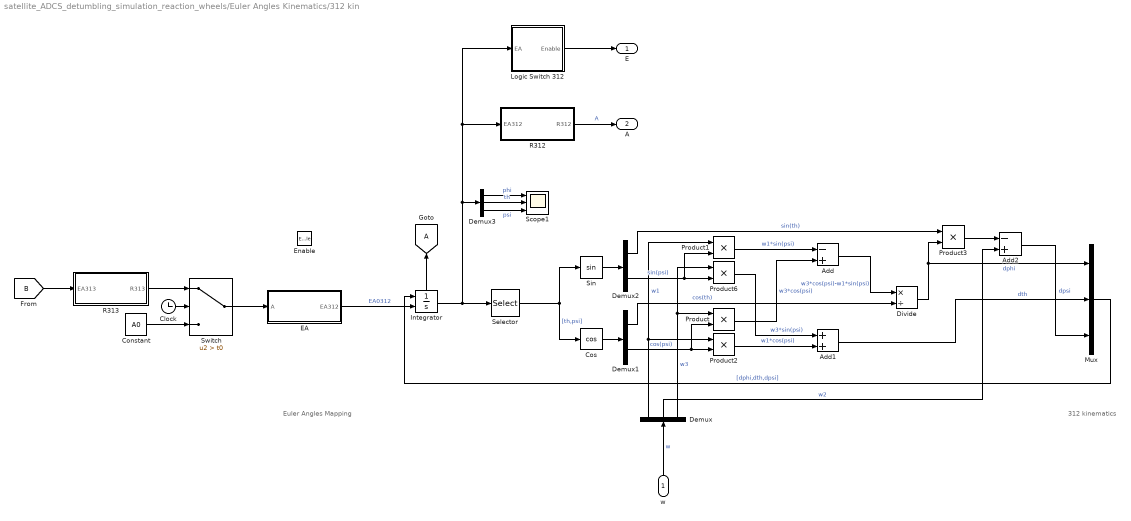
== system satellite_ADCS_detumbling_simulation_reaction_wheels/Euler Angles Kinematics/312 kin ==
  note: Euler Angles Mapping
  note: 312 kinematics
  w : Inport
  Enable : EnablePort  StatesWhenEnabling=reset
  Add : Sum  Inputs=-+
  Add1 : Sum
  Add2 : Sum  Inputs=-+
  Clock : Clock
  Constant : Constant  Value=A0
  Cos : Trigonometry  Operator=cos
  Demux : Demux  Outputs=3
  Demux1 : Demux  Outputs=2
  Demux2 : Demux  Outputs=2
  Demux3 : Demux  Outputs=3
  Divide : Product  Inputs=*/
  EA : Subsystem
  Goto : Goto  TagVisibility=global
  Integrator : Integrator  InitialConditionSource=external  WrapState=on  WrappedStateUpperValue=2*pi  WrappedStateLowerValue=0  ShowStatePort=on
  Logic Switch 312 : Subsystem
  Mux : Mux  Inputs=3
  Product{,1..3,6} (5 alike) : Product
  R312 : Subsystem
  R313 : Subsystem
  Scope1 : Scope  NumInputPorts=3
  Selector : Selector  InputPortWidth=3  IndexOptions=Index vector (dialog)  Indices=[2 3]  OutputSizes=1
  Sin : Trigonometry
  Switch : Switch  Criteria=u2 > Threshold  Threshold=t0  SaturateOnIntegerOverflow=off  InputSameDT=off
  E : Outport
  A : Outport  Port=2
  wires:
  Demux/2 -> Add2/2  "w2"
  Product1/1 -> Add/1  "w1*sin(psi)"
  w/1 -> Demux/1  "w"
  Product2/1 -> Add1/2  "w1*cos(psi)"
  Demux2/1 -> Product3/1  "sin(th)"
  Selector/1 -> Cos/1, Sin/1  "[th,psi]"
  Demux2/2 -> Product1/2, Product6/2  "sin(psi)"
  Sin/1 -> Demux2/1
  Demux/3 -> Product6/1, Product/1  "w3"
  EA/1(EA312) -> Integrator/2  "EA0312"
  Cos/1 -> Demux1/1
  Demux/1 -> Product1/1, Product2/1  "w1"
  Add2/1 -> Mux/3  "dpsi"
  Mux/1 -> Integrator/1  "[dphi,dth,dpsi]"
  Product/1 -> Add/2  "w3*cos(psi)"
  Divide/1 -> Product3/2, Mux/1  "dphi"
  Product6/1 -> Add1/1  "w3*sin(psi)"
  R312/1(R312) -> A/1  "A"
  Constant/1 -> Switch/3
  Product3/1 -> Add2/1
  Logic Switch 312/1(Enable) -> E/1
  Clock/1 -> Switch/2
  Add/1 -> Divide/1  "w3*cos(psi)-w1*sin(psi)"
  Demux1/2 -> Product/2, Product2/2  "cos(psi)"
  Add1/1 -> Mux/2  "dth"
  Demux1/1 -> Divide/2  "cos(th)"
  Switch/1 -> EA/1(A)
  Integrator/State -> Goto/1
  [B] -> R313/1(EA313)
  R313/1(R313) -> Switch/1
  Demux3/1 -> Scope1/1  "phi"
  Demux3/3 -> Scope1/3  "psi"
  Integrator/1 -> Demux3/1, R312/1(EA312), Logic Switch 312/1(EA), Selector/1
  Demux3/2 -> Scope1/2  "th"

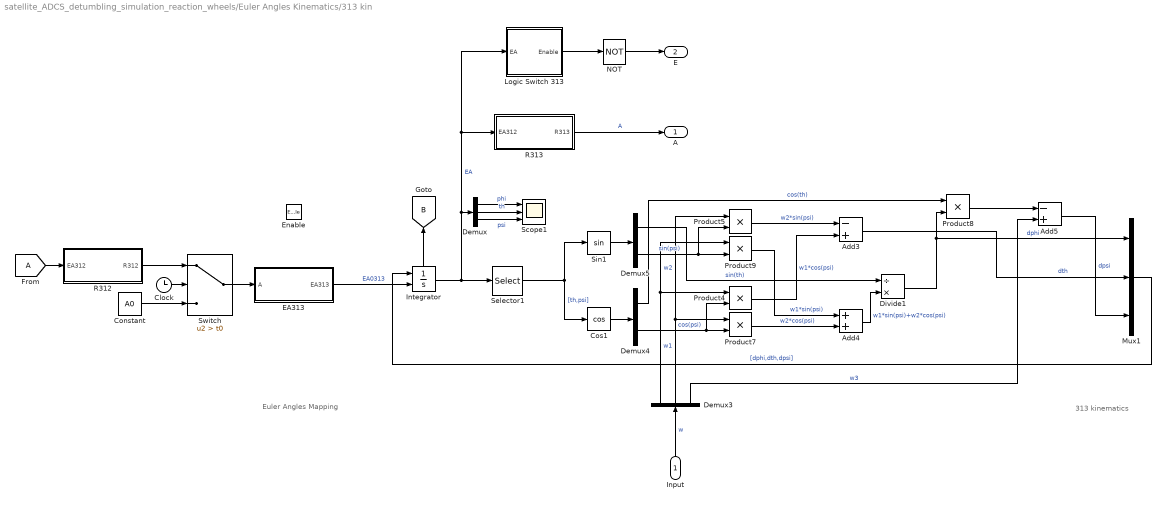
== system satellite_ADCS_detumbling_simulation_reaction_wheels/Euler Angles Kinematics/313 kin ==
  note: 313 kinematics
  note: Euler Angles Mapping
  Input : Inport
  Enable : EnablePort  StatesWhenEnabling=reset
  Add3 : Sum  Inputs=-+
  Add4 : Sum
  Add5 : Sum  Inputs=-+
  Clock : Clock
  Constant : Constant  Value=A0
  Cos1 : Trigonometry  Operator=cos
  Demux : Demux  Outputs=3
  Demux3 : Demux  Outputs=3
  Demux4 : Demux  Outputs=2
  Demux5 : Demux  Outputs=2
  Divide1 : Product  Inputs=/*
  EA313 : Subsystem
  From : From  TagVisibility=global
  Integrator : Integrator  InitialConditionSource=external  WrapState=on  WrappedStateUpperValue=2*pi  WrappedStateLowerValue=0  ShowStatePort=on
  Logic Switch 313 : Subsystem
  Mux1 : Mux  Inputs=3
  NOT : Logic  Operator=NOT  AllPortsSameDT=off  OutDataTypeStr=boolean
  Product{4..5,7..9} (5 alike) : Product
  R312 : Subsystem
  R313 : Subsystem
  Scope1 : Scope  NumInputPorts=3
  Selector1 : Selector  InputPortWidth=3  IndexOptions=Index vector (dialog)  Indices=[2 3]  OutputSizes=1
  Sin1 : Trigonometry
  Switch : Switch  Criteria=u2 > Threshold  Threshold=t0  SaturateOnIntegerOverflow=off  InputSameDT=off
  A : Outport
  E : Outport  Port=2
  tag scope: B=global
  wires:
  Selector1/1 -> Cos1/1, Sin1/1  "[th,psi]"
  Add4/1 -> Divide1/2  "w1*sin(psi)+w2*cos(psi)"
  EA313/1(EA313) -> Integrator/2  "EA0313"
  Demux5/2 -> Product5/2, Product9/2  "sin(psi)"
  Demux4/1 -> Product8/1  "cos(th)"
  Add3/1 -> Mux1/2  "dth"
  R313/1(R313) -> A/1  "A"
  Integrator/1 -> Demux/1, R313/1(EA312), Logic Switch 313/1(EA), Selector1/1  "EA"
  Cos1/1 -> Demux4/1
  Input/1 -> Demux3/1  "w"
  Sin1/1 -> Demux5/1
  Demux3/1 -> Product9/1, Product4/1  "w1"
  Divide1/1 -> Mux1/1, Product8/2  "dphi"
  Product4/1 -> Add3/2  "w1*cos(psi)"
  Product7/1 -> Add4/2  "w2*cos(psi)"
  Product9/1 -> Add4/1  "w1*sin(psi)"
  Add5/1 -> Mux1/3  "dpsi"
  Logic Switch 313/1(Enable) -> NOT/1
  Demux3/3 -> Add5/2  "w3"
  Product8/1 -> Add5/1
  Demux3/2 -> Product5/1, Product7/1  "w2"
  Product5/1 -> Add3/1  "w2*sin(psi)"
  Demux5/1 -> Divide1/1  "sin(th)"
  Demux4/2 -> Product4/2, Product7/2  "cos(psi)"
  Mux1/1 -> Integrator/1  "[dphi,dth,dpsi]"
  NOT/1 -> E/1
  From/1 -> R312/1(EA312)
  Integrator/State -> [B]
  Demux/1 -> Scope1/1  "phi"
  Demux/2 -> Scope1/2  "th"
  Demux/3 -> Scope1/3  "psi"
  Constant/1 -> Switch/3
  Clock/1 -> Switch/2
  Switch/1 -> EA313/1(A)
  R312/1(R312) -> Switch/1

== system satellite_ADCS_detumbling_simulation_reaction_wheels/Euler Angles Kinematics/Initial Conditions ==
  S : Inport
  Clock : Clock
  Constant : Constant  Value=E
  Switch : Switch  Criteria=u2 > Threshold  SaturateOnIntegerOverflow=off  InputSameDT=off
  E : Outport
  wires:
  Switch/1 -> E/1
  Clock/1 -> Switch/2
  Constant/1 -> Switch/3
  S/1 -> Switch/1

== system satellite_ADCS_detumbling_simulation_reaction_wheels/Pointing Control/Manual Control ==
  Constant : Constant
  Constant1 : Constant  Value=0
  On : Outport
  Off : Outport  Port=2
  wires:
  Constant/1 -> On/1
  Constant1/1 -> Off/1
